simulink model "a"  (R2019a)
settings: Solver=VariableStepAuto  StartTime=0.0  StopTime=1000  RelTol=1e-3
values from neighbouring files (symbols this model uses):
  o_m_a_d_d_c = [10 15 20 25 30;100 150 300 1 1;1 1 1 1 1]    [EventBasedEntityGenerationExample.m]
undefined symbols (not defined in the file or in its folder): m, n
settings Model: Creator=arsineh  LastModifiedBy=arsineh

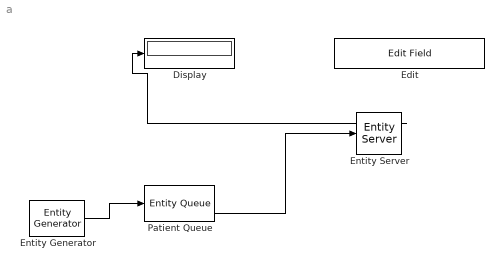
== system a ==
  Display : Display
  Edit : EditField  LabelPosition=Hide  ShowInitialText=on  Alignment=Center
  Entity Generator : EntityGenerator  OutputPortMessageModes=m  EntityType=Structured  EntityTypeName=Entity
  Entity Server : EntityServer  InputPortMessageModes=m  OutputPortMessageModes=n,m  Capacity=o_m_a_d_d_c(2,3)  ServiceTimeValue=10000  NumberEntitiesInBlock=on
      settings: OutputPortMap=o1,o9
  Patient Queue : EntityQueue  InputPortMessageModes=m  OutputPortMessageModes=n,n,m  Capacity=10  NumberEntitiesInBlock=on  AverageWait=on
      settings: OutputPortMap=o1,o2,o5
  wires:
  Entity Generator/1 -> Patient Queue/1
  Patient Queue/3 -> Entity Server/1
  Entity Server/1 -> Display/1
